simulink model "EnableDemo"  (R2014a)
settings: Solver=ode45  StartTime=0.0  StopTime=10.0  RelTol=1e-3
settings Model: Creator=李广文  LastModifiedBy=李广文

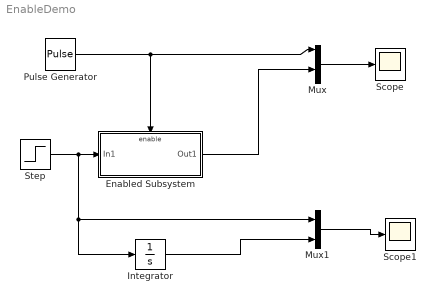
== system EnableDemo ==
  Enabled Subsystem : Subsystem  TreatAsAtomicUnit=on
  Integrator : Integrator
  Mux : Mux
  Mux1 : Mux  Inputs=2
  Pulse Generator : DiscretePulseGenerator  PulseType=Time based  Period=3  PulseWidth=50
  Scope : Scope
      settings: YMin=-2  YMax=2
  Scope1 : Scope
      settings: YMin=-2  YMax=2
  Step : Step  SampleTime=0
  wires:
  Pulse Generator/1 -> Mux/1, Enabled Subsystem/Enable
  Mux/1 -> Scope/1
  Step/1 -> Mux1/1, Integrator/1, Enabled Subsystem/1(In1)
  Integrator/1 -> Mux1/2
  Mux1/1 -> Scope1/1
  Enabled Subsystem/1(Out1) -> Mux/3

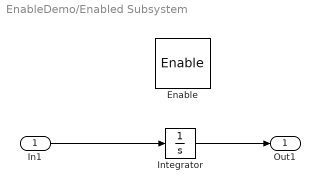
== system EnableDemo/Enabled Subsystem ==
  In1 : Inport
  Enable : EnablePort
  Integrator : Integrator
  Out1 : Outport
  wires:
  In1/1 -> Integrator/1
  Integrator/1 -> Out1/1
